simulink model "DynoController_Rev1"  (Simulink 7.7)
settings: Solver=FixedStepDiscrete  StartTime=0.0  StopTime=10.0  RelTol=1e-3
PreLoadFcn:
  | try, eval([bdroot '_setup']); catch, eval('model_setup', ''); end
InitFcn:
  | try, eval([bdroot '_setup']); catch, eval('model_setup', ''); end
undefined symbols (not defined in the file or in its folder): ECU555, motohawk_build_version, motohawk_trunc_name, motohawk_vardec_config_group, motohawk_vardec_path
libraries: MotoHawk_lib x160, MotoHawk_VDOGauge_lib x7, motohawk_annotations_lib x6, simulink x4, motohawk_control_primitives_lib x3
(part 3 of 3)

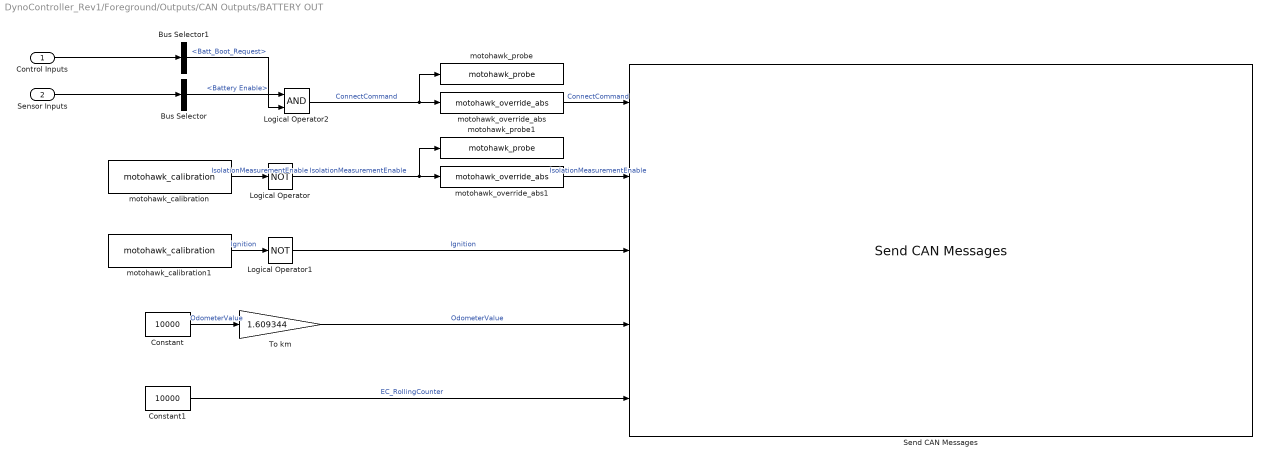
== system DynoController_Rev1/Foreground/Outputs/CAN Outputs/BATTERY OUT ==
  Control Inputs : Inport
  Sensor Inputs : Inport  Port=2
  Bus Selector : BusSelector  OutputSignals=Analog Inputs.Battery Enable
  Bus Selector1 : BusSelector  OutputSignals=Battery.Batt_Boot_Request
  Constant : Constant  Value=10000
  Constant1 : Constant  Value=10000
  Logical Operator : Logic  Operator=NOT  AllPortsSameDT=off  OutDataTypeStr=boolean
  Logical Operator1 : Logic  Operator=NOT  AllPortsSameDT=off  OutDataTypeStr=boolean
  Logical Operator2 : Logic  AllPortsSameDT=off  OutDataTypeStr=boolean
  Send CAN Messages : MotoHawk_lib/CAN Blocks/Send CAN Messages  bus=-2  nam=['CAN_' num2str(1)]  msgl=CANTx_BATTERY_2F0  pace=5  labelwires=on
  To km : Gain  Gain=1.609344
  motohawk_calibration : MotoHawk_lib/Calibration & Probing Blocks/motohawk_calibration  nam='Batt_Isolation_det_Cal'  val=1  storage=Calibration NV  show_more=off  name_source=Use Parameter  data_type=Inherit from 'Default Value'  read_level=1  write_level=1  ovr_cals=on  view_as=Number  enum_struct={'Disabled', 'Enabled'}  vector_style=Wide Row  use_help_units=off  help=''  units=''  use_header_enum=off  row_header_enum={}  col_header_enum={}  use_min_max=off  min_val=-inf  max_val=inf  use_precision=off  precision=''  gain=1  offset=0  exp=1  use_mototune_group=off  mototune_group=motohawk_vardec_path(gcb)
  motohawk_calibration1 : MotoHawk_lib/Calibration & Probing Blocks/motohawk_calibration  nam='Batt_Ign_Cal'  val=1  storage=Calibration NV  show_more=off  name_source=Use Parameter  data_type=Inherit from 'Default Value'  read_level=1  write_level=1  ovr_cals=on  view_as=Number  enum_struct={'Disabled', 'Enabled'}  vector_style=Wide Row  use_help_units=off  help=''  units=''  use_header_enum=off  row_header_enum={}  col_header_enum={}  use_min_max=off  min_val=-inf  max_val=inf  use_precision=off  precision=''  gain=1  offset=0  exp=1  use_mototune_group=off  mototune_group=motohawk_vardec_path(gcb)
  motohawk_override_abs : MotoHawk_lib/Calibration & Probing Blocks/motohawk_override_abs  SystemSampleTime=-1  parent_name='Batt_Connect_Cmd_ovr'  parent_val=0  show_more=on  name_source=Use Parameter  parent_read_level=1  parent_override_level=1  view_as=Number  enum_struct={'Disabled', 'Enabled'}  use_help_units=off  parent_help=''  parent_units=''  use_min_max=on  parent_min=0  parent_max=4  use_precision=off  parent_precision=''  parent_gain=1  parent_offset=0  parent_exp=1  use_mototune_group=off  parent_group=motohawk_vardec_path(gcb)
  motohawk_override_abs1 : MotoHawk_lib/Calibration & Probing Blocks/motohawk_override_abs  SystemSampleTime=-1  parent_name='Isolation_Measure_Enable_ovr'  parent_val=0  show_more=on  name_source=Use Parameter  parent_read_level=1  parent_override_level=1  view_as=Number  enum_struct={'Disabled', 'Enabled'}  use_help_units=off  parent_help=''  parent_units=''  use_min_max=on  parent_min=0  parent_max=3  use_precision=off  parent_precision=''  parent_gain=1  parent_offset=0  parent_exp=1  use_mototune_group=off  parent_group=motohawk_vardec_path(gcb)
  motohawk_probe : MotoHawk_lib/Calibration & Probing Blocks/motohawk_probe  nam='Batt_Connect_Cmd_Probe'  show_more=on  name_source=Use Parameter  read_level=1  view_as=Number  enum_struct={'Disabled', 'Enabled'}  vector_style=Wide Row  use_help_units=off  help=''  units=''  use_header_enum=off  row_header_enum={}  col_header_enum={}  use_precision=off  precision=''  gain=1  offset=0  exp=1  use_mototune_group=off  mototune_group=motohawk_vardec_path(gcb)
  motohawk_probe1 : MotoHawk_lib/Calibration & Probing Blocks/motohawk_probe  nam='Isolation_Measure_Enable_Probe'  show_more=on  name_source=Use Parameter  read_level=1  view_as=Number  enum_struct={'Disabled', 'Enabled'}  vector_style=Wide Row  use_help_units=off  help=''  units=''  use_header_enum=off  row_header_enum={}  col_header_enum={}  use_precision=off  precision=''  gain=1  offset=0  exp=1  use_mototune_group=off  mototune_group=motohawk_vardec_path(gcb)
  wires:
  motohawk_calibration/1 -> Logical Operator/1  "IsolationMeasurementEnable"
  motohawk_calibration1/1 -> Logical Operator1/1  "Ignition"
  Logical Operator2/1 -> motohawk_override_abs/1, motohawk_probe/1  "ConnectCommand"
  motohawk_override_abs/1 -> Send CAN Messages/1  "ConnectCommand"
  Logical Operator/1 -> motohawk_override_abs1/1, motohawk_probe1/1  "IsolationMeasurementEnable"
  motohawk_override_abs1/1 -> Send CAN Messages/2  "IsolationMeasurementEnable"
  Constant/1 -> To km/1  "OdometerValue"
  Logical Operator1/1 -> Send CAN Messages/3  "Ignition"
  To km/1 -> Send CAN Messages/4  "OdometerValue"
  Constant1/1 -> Send CAN Messages/5  "EC_RollingCounter"
  Sensor Inputs/1 -> Bus Selector/1
  Control Inputs/1 -> Bus Selector1/1
  Bus Selector/1 -> Logical Operator2/1  "<Battery Enable>"
  Bus Selector1/1 -> Logical Operator2/2  "<Batt_Boot_Request>"

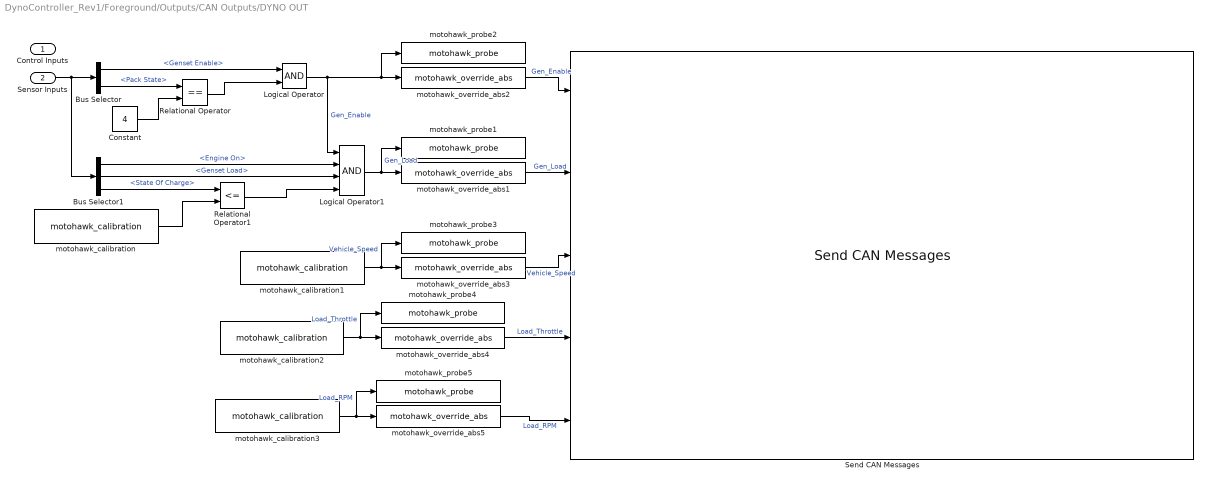
== system DynoController_Rev1/Foreground/Outputs/CAN Outputs/DYNO OUT ==
  Control Inputs : Inport
  Sensor Inputs : Inport  Port=2
  Bus Selector : BusSelector  OutputSignals=Analog Inputs.Genset Enable,CAN Inputs.BATTERY.Pack State
  Bus Selector1 : BusSelector  OutputSignals=CAN Inputs.DYNO.Engine On,Analog Inputs.Genset Load,CAN Inputs.BATTERY.State Of Charge
  Constant : Constant  Value=4
  Logical Operator : Logic  AllPortsSameDT=off  OutDataTypeStr=boolean
  Logical Operator1 : Logic  Inputs=4  AllPortsSameDT=off  OutDataTypeStr=boolean
  Relational Operator : RelationalOperator  Operator===  OutDataTypeStr=boolean
  Relational Operator1 : RelationalOperator  Operator=<=  OutDataTypeStr=boolean
  Send CAN Messages : MotoHawk_lib/CAN Blocks/Send CAN Messages  bus=-2  nam=['CAN_' num2str(1)]  msgl=CANTx_112_210  pace=5  labelwires=on
  motohawk_calibration : MotoHawk_lib/Calibration & Probing Blocks/motohawk_calibration  nam='SOC_Off_Pt'  val=80  storage=Calibration  show_more=off  name_source=Use Parameter  data_type=Inherit from 'Default Value'  read_level=1  write_level=1  ovr_cals=on  view_as=Number  enum_struct={'Disabled', 'Enabled'}  vector_style=Wide Row  use_help_units=off  help=''  units=''  use_header_enum=off  row_header_enum={}  col_header_enum={}  use_min_max=off  min_val=-inf  max_val=inf  use_precision=off  precision=''  gain=1  offset=0  exp=1  use_mototune_group=off  mototune_group=motohawk_vardec_path(gcb)
  motohawk_calibration1 : MotoHawk_lib/Calibration & Probing Blocks/motohawk_calibration  nam='Vehicle_Speed'  val=0  storage=Calibration  show_more=off  name_source=Use Parameter  data_type=Inherit from 'Default Value'  read_level=1  write_level=1  ovr_cals=on  view_as=Number  enum_struct={'Disabled', 'Enabled'}  vector_style=Wide Row  use_help_units=off  help=''  units=''  use_header_enum=off  row_header_enum={}  col_header_enum={}  use_min_max=off  min_val=-inf  max_val=inf  use_precision=off  precision=''  gain=1  offset=0  exp=1  use_mototune_group=off  mototune_group=motohawk_vardec_path(gcb)
  motohawk_calibration2 : MotoHawk_lib/Calibration & Probing Blocks/motohawk_calibration  nam='Load_Throttle'  val=0  storage=Display  show_more=off  name_source=Use Parameter  data_type=Inherit from 'Default Value'  read_level=1  write_level=1  ovr_cals=on  view_as=Number  enum_struct={'Disabled', 'Enabled'}  vector_style=Wide Row  use_help_units=off  help=''  units=''  use_header_enum=off  row_header_enum={}  col_header_enum={}  use_min_max=off  min_val=-inf  max_val=inf  use_precision=off  precision=''  gain=1  offset=0  exp=1  use_mototune_group=off  mototune_group=motohawk_vardec_path(gcb)
  motohawk_calibration3 : MotoHawk_lib/Calibration & Probing Blocks/motohawk_calibration  nam='Load_RPM'  val=0  storage=Display  show_more=off  name_source=Use Parameter  data_type=Inherit from 'Default Value'  read_level=1  write_level=1  ovr_cals=on  view_as=Number  enum_struct={'Disabled', 'Enabled'}  vector_style=Wide Row  use_help_units=off  help=''  units=''  use_header_enum=off  row_header_enum={}  col_header_enum={}  use_min_max=off  min_val=-inf  max_val=inf  use_precision=off  precision=''  gain=1  offset=0  exp=1  use_mototune_group=off  mototune_group=motohawk_vardec_path(gcb)
  motohawk_override_abs1 : MotoHawk_lib/Calibration & Probing Blocks/motohawk_override_abs  SystemSampleTime=-1  parent_name='Gen_Load_Ovr'  parent_val=0  show_more=off  name_source=Use Parameter  parent_read_level=1  parent_override_level=1  view_as=Number  enum_struct={'Disabled', 'Enabled'}  use_help_units=off  parent_help=''  parent_units=''  use_min_max=off  parent_min=-inf  parent_max=inf  use_precision=off  parent_precision=''  parent_gain=1  parent_offset=0  parent_exp=1  use_mototune_group=off  parent_group=motohawk_vardec_path(gcb)
  motohawk_override_abs2 : MotoHawk_lib/Calibration & Probing Blocks/motohawk_override_abs  SystemSampleTime=-1  parent_name='Gen_Enable_Ovr'  parent_val=0  show_more=off  name_source=Use Parameter  parent_read_level=1  parent_override_level=1  view_as=Number  enum_struct={'Disabled', 'Enabled'}  use_help_units=off  parent_help=''  parent_units=''  use_min_max=off  parent_min=-inf  parent_max=inf  use_precision=off  parent_precision=''  parent_gain=1  parent_offset=0  parent_exp=1  use_mototune_group=off  parent_group=motohawk_vardec_path(gcb)
  motohawk_override_abs3 : MotoHawk_lib/Calibration & Probing Blocks/motohawk_override_abs  SystemSampleTime=-1  parent_name='Vehicle_Speed_Ovr'  parent_val=0  show_more=off  name_source=Use Parameter  parent_read_level=1  parent_override_level=1  view_as=Number  enum_struct={'Disabled', 'Enabled'}  use_help_units=off  parent_help=''  parent_units=''  use_min_max=off  parent_min=-inf  parent_max=inf  use_precision=off  parent_precision=''  parent_gain=1  parent_offset=0  parent_exp=1  use_mototune_group=off  parent_group=motohawk_vardec_path(gcb)
  motohawk_override_abs4 : MotoHawk_lib/Calibration & Probing Blocks/motohawk_override_abs  SystemSampleTime=-1  parent_name='Load_Throttle_Ovr'  parent_val=0  show_more=off  name_source=Use Parameter  parent_read_level=1  parent_override_level=1  view_as=Number  enum_struct={'Disabled', 'Enabled'}  use_help_units=off  parent_help=''  parent_units=''  use_min_max=off  parent_min=-inf  parent_max=inf  use_precision=off  parent_precision=''  parent_gain=1  parent_offset=0  parent_exp=1  use_mototune_group=off  parent_group=motohawk_vardec_path(gcb)
  motohawk_override_abs5 : MotoHawk_lib/Calibration & Probing Blocks/motohawk_override_abs  SystemSampleTime=-1  parent_name='Load_RPM_Ovr'  parent_val=0  show_more=off  name_source=Use Parameter  parent_read_level=1  parent_override_level=1  view_as=Number  enum_struct={'Disabled', 'Enabled'}  use_help_units=off  parent_help=''  parent_units=''  use_min_max=off  parent_min=-inf  parent_max=inf  use_precision=off  parent_precision=''  parent_gain=1  parent_offset=0  parent_exp=1  use_mototune_group=off  parent_group=motohawk_vardec_path(gcb)
  motohawk_probe1 : MotoHawk_lib/Calibration & Probing Blocks/motohawk_probe  nam='Gen_Load_Prb'  show_more=off  name_source=Use Parameter  read_level=1  view_as=Number  enum_struct={'Disabled', 'Enabled'}  vector_style=Wide Row  use_help_units=off  help=''  units=''  use_header_enum=off  row_header_enum={}  col_header_enum={}  use_precision=off  precision=''  gain=1  offset=0  exp=1  use_mototune_group=off  mototune_group=motohawk_vardec_path(gcb)
  motohawk_probe2 : MotoHawk_lib/Calibration & Probing Blocks/motohawk_probe  nam='Gen_Enable_Prb'  show_more=off  name_source=Use Parameter  read_level=1  view_as=Number  enum_struct={'Disabled', 'Enabled'}  vector_style=Wide Row  use_help_units=off  help=''  units=''  use_header_enum=off  row_header_enum={}  col_header_enum={}  use_precision=off  precision=''  gain=1  offset=0  exp=1  use_mototune_group=off  mototune_group=motohawk_vardec_path(gcb)
  motohawk_probe3 : MotoHawk_lib/Calibration & Probing Blocks/motohawk_probe  nam='Vehicle_Speed_Prb'  show_more=off  name_source=Use Parameter  read_level=1  view_as=Number  enum_struct={'Disabled', 'Enabled'}  vector_style=Wide Row  use_help_units=off  help=''  units=''  use_header_enum=off  row_header_enum={}  col_header_enum={}  use_precision=off  precision=''  gain=1  offset=0  exp=1  use_mototune_group=off  mototune_group=motohawk_vardec_path(gcb)
  motohawk_probe4 : MotoHawk_lib/Calibration & Probing Blocks/motohawk_probe  nam='Load_Throttle_Prb'  show_more=off  name_source=Use Parameter  read_level=1  view_as=Number  enum_struct={'Disabled', 'Enabled'}  vector_style=Wide Row  use_help_units=off  help=''  units=''  use_header_enum=off  row_header_enum={}  col_header_enum={}  use_precision=off  precision=''  gain=1  offset=0  exp=1  use_mototune_group=off  mototune_group=motohawk_vardec_path(gcb)
  motohawk_probe5 : MotoHawk_lib/Calibration & Probing Blocks/motohawk_probe  nam='Load_RPM_Prb'  show_more=off  name_source=Use Parameter  read_level=1  view_as=Number  enum_struct={'Disabled', 'Enabled'}  vector_style=Wide Row  use_help_units=off  help=''  units=''  use_header_enum=off  row_header_enum={}  col_header_enum={}  use_precision=off  precision=''  gain=1  offset=0  exp=1  use_mototune_group=off  mototune_group=motohawk_vardec_path(gcb)
  wires:
  motohawk_override_abs2/1 -> Send CAN Messages/1  "Gen_Enable"
  motohawk_override_abs1/1 -> Send CAN Messages/2  "Gen_Load"
  motohawk_override_abs3/1 -> Send CAN Messages/3  "Vehicle_Speed"
  Logical Operator/1 -> motohawk_override_abs2/1, motohawk_probe2/1, Logical Operator1/1  "Gen_Enable"
  Sensor Inputs/1 -> Bus Selector/1, Bus Selector1/1
  Bus Selector/1 -> Logical Operator/1  "<Genset Enable>"
  Bus Selector/2 -> Relational Operator/1  "<Pack State>"
  Constant/1 -> Relational Operator/2
  Relational Operator/1 -> Logical Operator/2
  Logical Operator1/1 -> motohawk_override_abs1/1, motohawk_probe1/1  "Gen_Load"
  Bus Selector1/1 -> Logical Operator1/2  "<Engine On>"
  Bus Selector1/2 -> Logical Operator1/3  "<Genset Load>"
  Bus Selector1/3 -> Relational Operator1/1  "<State Of Charge>"
  motohawk_calibration/1 -> Relational Operator1/2
  Relational Operator1/1 -> Logical Operator1/4
  motohawk_calibration1/1 -> motohawk_override_abs3/1, motohawk_probe3/1  "Vehicle_Speed"
  motohawk_calibration2/1 -> motohawk_override_abs4/1, motohawk_probe4/1  "Load_Throttle"
  motohawk_calibration3/1 -> motohawk_override_abs5/1, motohawk_probe5/1  "Load_RPM"
  motohawk_override_abs4/1 -> Send CAN Messages/4  "Load_Throttle"
  motohawk_override_abs5/1 -> Send CAN Messages/5  "Load_RPM"

== system DynoController_Rev1/Foreground/Outputs/Guages/Time Since Key On ==
  Constant : Constant  Value=true
  Time Since Enabled (With Input)2 : motohawk_control_primitives_lib/Time Since Enabled (With Input)1  SystemSampleTime=-1  nam='TimeSinceKeyOnTimer'  samp_time=-1  init=0  upperlim=16000
  motohawk_probe : MotoHawk_lib/Calibration & Probing Blocks/motohawk_probe  nam='TimeSinceKeyOn'  show_more=on  name_source=Use Parameter  read_level=1  view_as=Number  enum_struct={'Disabled', 'Enabled'}  vector_style=Wide Row  use_help_units=off  help=''  units=''  use_header_enum=off  row_header_enum={}  col_header_enum={}  use_precision=off  precision=''  gain=1  offset=0  exp=1  use_mototune_group=on  mototune_group=motohawk_vardec_path(gcb)
  Time : Outport
  wires:
  Constant/1 -> Time Since Enabled (With Input)2/1
  Time Since Enabled (With Input)2/1 -> Time/1, motohawk_probe/1

== system DynoController_Rev1/Main Power Relay/Background/Delay/MotoHawk S-R Flip-Flop ==
  note: MotoHawk S-R Flip-Flop
  S : Inport
  R : Inport  Port=2
  Logical Operator : Logic  Operator=OR  OutDataTypeStr=boolean
  Logical Operator1 : Logic  Operator=NOT  OutDataTypeStr=boolean
  Logical Operator2 : Logic  OutDataTypeStr=boolean
  Logical Operator3 : Logic  Operator=NOT  OutDataTypeStr=boolean
  Signal Specification : SignalSpecification  OutDataTypeStr=boolean
  Signal Specification1 : SignalSpecification  OutDataTypeStr=boolean
  Unit Delay : UnitDelay  X0=ic_bool  SampleTime=-1
  Q : Outport
  !Q : Outport  Port=2
  wires:
  Logical Operator3/1 -> !Q/1
  R/1 -> Signal Specification/1
  S/1 -> Signal Specification1/1
  Signal Specification1/1 -> Logical Operator/2
  Signal Specification/1 -> Logical Operator1/1
  Logical Operator2/1 -> Q/1, Unit Delay/1, Logical Operator3/1
  Unit Delay/1 -> Logical Operator/1
  Logical Operator/1 -> Logical Operator2/1
  Logical Operator1/1 -> Logical Operator2/2

== stateflow chart Foreground/Control/Vehicle Run/Stop Determination/Chart ==
  state Initial
    during:
    Vehicle_Enable=false
    Vehicle_Ready=false
    Torque_Enable=false
    Keyed_Relay=true;
  state Batterybootup
    during:
    Vehicle_Enable=true
    Vehicle_Ready=false
    Torque_Enable=false
    Keyed_Relay=true;
  state Charging_and_Temp
    during:
    Vehicle_Enable=true
    Vehicle_Ready=true
    Torque_Enable=false
    Keyed_Relay=true;
  state Normal_Operation
    during:
    Vehicle_Enable=true
    Vehicle_Ready=true
    Torque_Enable=true
    Keyed_Relay=true;
  state Shutdown_Sequence
    during:
    Vehicle_Enable=false
    Vehicle_Ready=false
    Torque_Enable=false
    Keyed_Relay=true;
  state Kill_Component_Keyed
    during:
    Vehicle_Enable=false
    Vehicle_Ready=false
    Torque_Enable=false
    Keyed_Relay=false;
  (default) -> Initial
  Initial -> Batterybootup [order 1] : [!Shutdown]
  Initial -> Shutdown_Sequence [order 2] : [Shutdown]
  Charging_and_Temp -> Normal_Operation [order 2] : [!Charging]
  Batterybootup -> Shutdown_Sequence [order 1] : [Shutdown]
  Charging_and_Temp -> Shutdown_Sequence [order 1] : [Shutdown]
  Normal_Operation -> Shutdown_Sequence [order 1] : [Shutdown]
  Normal_Operation -> Charging_and_Temp [order 2] : [Charging]
  Shutdown_Sequence -> Kill_Component_Keyed : [!Batt_Contactor_Status]
  Batterybootup -> Charging_and_Temp [order 2] : [Batt_Load_Enable]
  data: Shutdown input boolean; Batt_Load_Enable input boolean; Vehicle_Enable output boolean; Vehicle_Ready output boolean; Torque_Enable output boolean; Keyed_Relay output boolean; Batt_Contactor_Status input boolean; Charging input boolean
